simulink model "visual_line_follower_with_debug"  (R2026a)
settings: Solver=FixedStepDiscrete  StopTime=40  FixedStep=MJ_StepTime  EnableMultiTasking=on
InitFcn:
  | run(fullfile(fileparts(get_param(bdroot,"FileName")),"runtime","init","configure_turtlebot3_visual_line_follower_paths.m"));
model workspace (MAT data in the model file):
  BaseLinearSpeed = 5
  BaseSpeedScale = 0.03
  Kd_Line = 0.35
  Ki_Line = 0
  Kp_Line = 5
  LocalPath_CurvatureGain = 0.04
  LocalPath_HeadingGain = 0.35
  LocalPath_LateralGain = 0.6
  LocalPath_LookaheadDistance = 0.2
  LocalPath_NumPoints = 30
  LocalPath_ROIFraction = 0.3
  MJ_StepTime = 0.002
  MJ_TargetLateralPosition = 0
  MaxAngularSpeed = 1.5
  MaxWheelSpeed = 7.9
  N_Line = 20
  OriginBot_ErrorScale = 500
  OriginBot_MaxSaturation = 0.3
  OriginBot_MinBrightness = 70
  OriginBot_MinPixels = 30
  OriginBot_ROIHeight = 45
  OriginBot_ROIStartFraction = 0.72
  SteeringSign = -1
  TB3_WheelRadius = 0.033
  TB3_WheelSeparation = 0.16
  Ts_Control = 0.05
  Ts_Vision = 0.05
  TurtleBot3MuJoCoMap = "complex"
  TurtleBot3MuJoCoScene = ""
values from neighbouring files (symbols this model uses):
  src = get_param(source, "PortHandles")    [add_local_path_to_visual_model.m]
undefined symbols (not defined in the file or in its folder): originbot_line_follower_debug_frame, originbot_sliding_window_path_generator
libraries: mjLib x1, slpidlib x1
settings Model: ExtModeTrigDuration=10000  Creator=HP  LastModifiedBy=kevin
settings SolverCC: PositivePriorityOrder=on
settings ConfigComp: CovMetricSettings=dswe

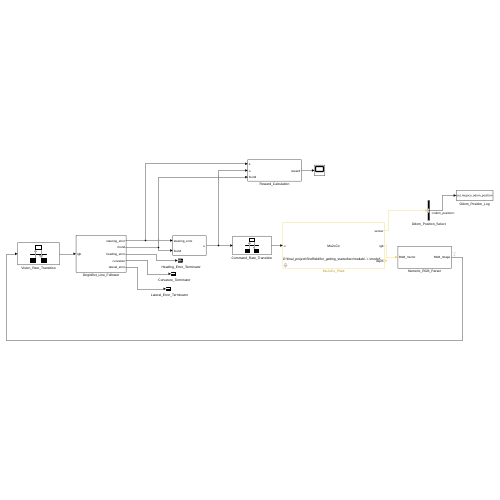
[thumbnail: Simulink's stored preview of the top-level diagram]
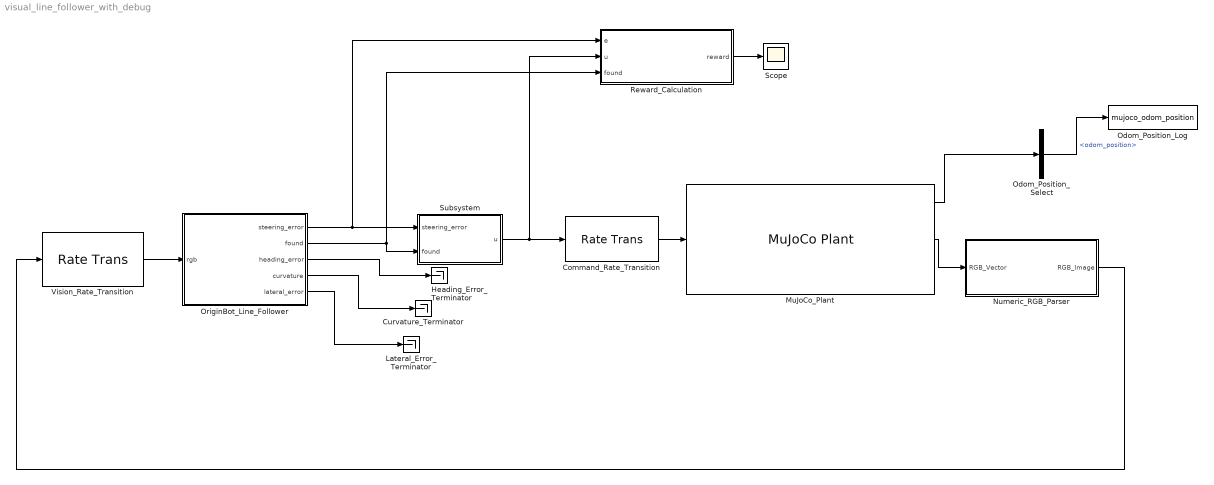
== system visual_line_follower_with_debug ==
  Command_Rate_Transition : RateTransition  OutPortSampleTime=MJ_StepTime
  Curvature_Terminator : Terminator
  Heading_Error_Terminator : Terminator
  Lateral_Error_Terminator : Terminator
  MuJoCo_Plant : mjLib/MuJoCo Plant  controlBus=[]  sensorBus=mj_bus_sensor_7979902499018342666  controlLength=[]  sensorLength=[]  rgbLength=[]  depthLength=[]  sampleTime=0.002  xmlFileRel=D:\final_project\Sheffield\for_getting_started\src\matlab\..\..\model\mujoco\turtlebot3\simple_camera_track_turtlebot3_burger_visual_scene.xml  xmlFile=D:\final_project\Sheffield\for_getting_started\src\matlab\..\..\model\mujoco\turtlebot3\simple_camera_track_turtlebot3_burger_visual_scene.xml  renderingType=Local  vsync=off  visualFPS=60  zoomLevel=1  znear=0.062275  zfar=311.3772  cameraSampleTime=Ts_Vision  rgbOutOption=on  depthOutOption=off  controlInterfaceType=Vector
      settings: SourceProductName=MuJoCo Simulator
  Numeric_RGB_Parser : Subsystem
  Odom_Position_Log : ToWorkspace  VariableName=mujoco_odom_position  SaveFormat=Timeseries  SampleTime=-1
  Odom_Position_Select : BusSelector  OutputSignals=odom_position
  OriginBot_Line_Follower : Subsystem
  Reward_Calculation : Subsystem
  Scope : Scope
      settings: ActiveDisplayYMinimum=-41.521611192700504  ActiveDisplayYMaximum=3.5588120226586528
  Subsystem : Subsystem
  Vision_Rate_Transition : RateTransition  OutPortSampleTime=Ts_Vision
  wires:
  Vision_Rate_Transition/1 -> OriginBot_Line_Follower/1(rgb)
  OriginBot_Line_Follower/1(steering_error) -> Reward_Calculation/1(e), Subsystem/1(steering_error)
  OriginBot_Line_Follower/3(heading_error) -> Heading_Error_Terminator/1
  OriginBot_Line_Follower/2(found) -> Reward_Calculation/3(found), Subsystem/2(found)
  OriginBot_Line_Follower/4(curvature) -> Curvature_Terminator/1
  OriginBot_Line_Follower/5(lateral_error) -> Lateral_Error_Terminator/1
  Subsystem/1(u) -> Reward_Calculation/2(u), Command_Rate_Transition/1
  Reward_Calculation/1(reward) -> Scope/1
  Command_Rate_Transition/1 -> MuJoCo_Plant/1
  MuJoCo_Plant/1 -> Odom_Position_Select/1
  MuJoCo_Plant/2 -> Numeric_RGB_Parser/1(RGB_Vector)
  Odom_Position_Select/1 -> Odom_Position_Log/1  "<odom_position>"
  Numeric_RGB_Parser/1(RGB_Image) -> Vision_Rate_Transition/1

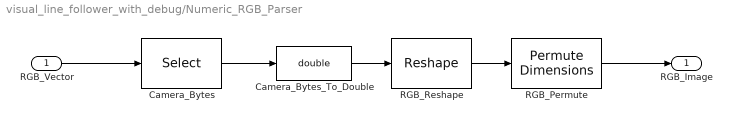
== system visual_line_follower_with_debug/Numeric_RGB_Parser ==
  RGB_Vector : Inport
  Camera_Bytes : Selector  InputPortWidth=921601  IndexOptions=Index vector (dialog)  Indices=1:921600  OutputSizes=1
  Camera_Bytes_To_Double : DataTypeConversion  OutDataTypeStr=double
  RGB_Permute : PermuteDimensions  Order=[3 2 1]
  RGB_Reshape : Reshape  OutputDimensionality=Customize  OutputDimensions=[3,640,480]
  RGB_Image : Outport
  wires:
  Camera_Bytes_To_Double/1 -> RGB_Reshape/1
  RGB_Permute/1 -> RGB_Image/1
  RGB_Reshape/1 -> RGB_Permute/1
  Camera_Bytes/1 -> Camera_Bytes_To_Double/1
  RGB_Vector/1 -> Camera_Bytes/1

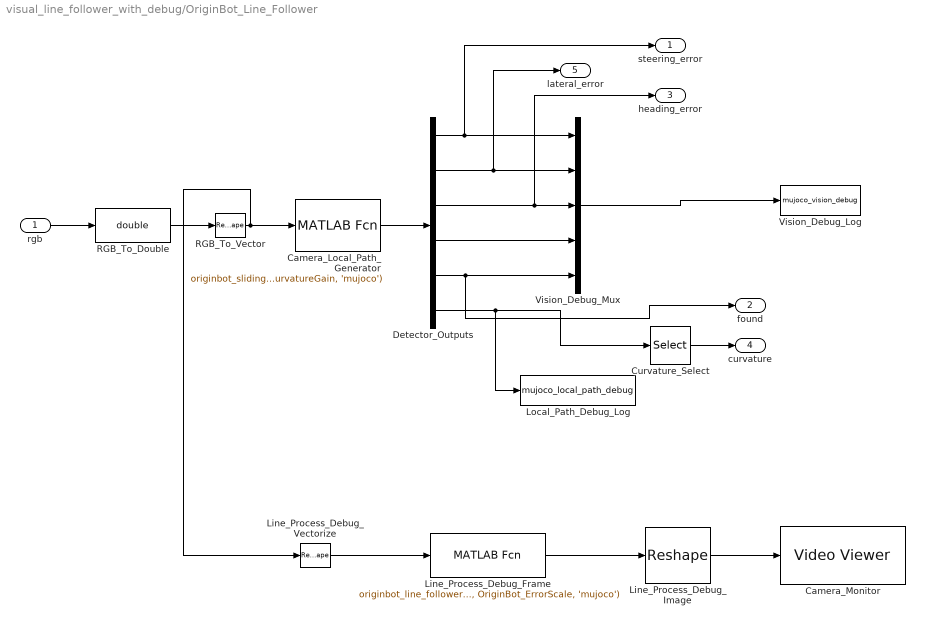
== system visual_line_follower_with_debug/OriginBot_Line_Follower ==
  rgb : Inport
  Camera_Local_Path_Generator : MATLABFcn  MATLABFcn=originbot_sliding_window_path_generator(u, LocalPath_ROIFraction, LocalPath_NumPoints, OriginBot_MinBrightness, OriginBot_MaxSaturation, OriginBot_MinPixels, OriginBot_ErrorScale, LocalPath_LookaheadDistance, LocalPath_LateralGain, LocalPath_HeadingGain, LocalPath_CurvatureGain, 'mujoco')  OutputDimensions=72  OutputSignalType=real  SampleTime=Ts_Vision
  Camera_Monitor : VideoViewer  FigPos=[402 652 810 551]
  Curvature_Select : Selector  InputPortWidth=67  IndexOptions=Index vector (dialog)  Indices=4  OutputSizes=1
  Detector_Outputs : Demux  Outputs=[1 1 1 1 1 67]
  Line_Process_Debug_Frame : MATLABFcn  MATLABFcn=originbot_line_follower_debug_frame(u, LocalPath_ROIFraction, LocalPath_NumPoints, OriginBot_MinBrightness, OriginBot_MaxSaturation, OriginBot_MinPixels, OriginBot_ErrorScale, 'mujoco')
  Line_Process_Debug_Image : Reshape  OutputDimensionality=Customize  OutputDimensions=[480,640,3]
  Line_Process_Debug_Vectorize : Reshape  OutputDimensionality=Column vector (2-D)
  Local_Path_Debug_Log : ToWorkspace  VariableName=mujoco_local_path_debug  SaveFormat=Timeseries  SampleTime=-1
  RGB_To_Double : DataTypeConversion  OutDataTypeStr=double
  RGB_To_Vector : Reshape  OutputDimensionality=Column vector (2-D)
  Vision_Debug_Log : ToWorkspace  VariableName=mujoco_vision_debug  SaveFormat=Timeseries  SampleTime=-1
  Vision_Debug_Mux : Mux  Inputs=5
  steering_error : Outport
  found : Outport  Port=2
  heading_error : Outport  Port=3
  curvature : Outport  Port=4
  lateral_error : Outport  Port=5
  wires:
  Vision_Debug_Mux/1 -> Vision_Debug_Log/1
  Detector_Outputs/1 -> steering_error/1, Vision_Debug_Mux/1
  Detector_Outputs/5 -> Vision_Debug_Mux/5, found/1
  Detector_Outputs/2 -> Vision_Debug_Mux/2, lateral_error/1
  Detector_Outputs/6 -> Curvature_Select/1, Local_Path_Debug_Log/1
  Detector_Outputs/3 -> heading_error/1, Vision_Debug_Mux/3
  Detector_Outputs/4 -> Vision_Debug_Mux/4
  RGB_To_Double/1 -> RGB_To_Vector/1
  RGB_To_Vector/1 -> Camera_Local_Path_Generator/1, Line_Process_Debug_Vectorize/1
  rgb/1 -> RGB_To_Double/1
  Camera_Local_Path_Generator/1 -> Detector_Outputs/1
  Curvature_Select/1 -> curvature/1
  Line_Process_Debug_Frame/1 -> Line_Process_Debug_Image/1
  Line_Process_Debug_Image/1 -> Camera_Monitor/1
  Line_Process_Debug_Vectorize/1 -> Line_Process_Debug_Frame/1

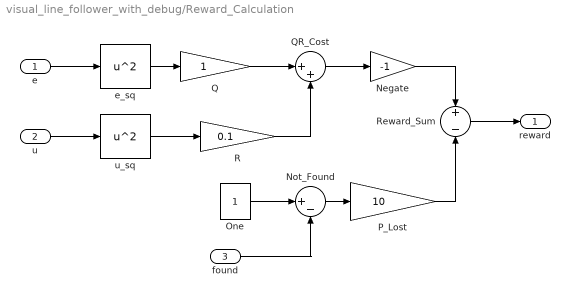
== system visual_line_follower_with_debug/Reward_Calculation ==
  e : Inport
  u : Inport  Port=2
  found : Inport  Port=3
  Negate : Gain  Gain=-1
  Not_Found : Sum  Inputs=|+-
  One : Constant
  P_Lost : Gain  Gain=10
  Q : Gain
  QR_Cost : Sum  Inputs=|++
  R : Gain  Gain=0.1
  Reward_Sum : Sum  Inputs=+-
  e_sq : Math  Operator=square
  u_sq : Math  Operator=square
  reward : Outport
  wires:
  Q/1 -> QR_Cost/1
  e/1 -> e_sq/1
  u/1 -> u_sq/1
  R/1 -> QR_Cost/2
  e_sq/1 -> Q/1
  u_sq/1 -> R/1
  One/1 -> Not_Found/1
  found/1 -> Not_Found/2
  QR_Cost/1 -> Negate/1
  Not_Found/1 -> P_Lost/1
  P_Lost/1 -> Reward_Sum/2
  Negate/1 -> Reward_Sum/1
  Reward_Sum/1 -> reward/1

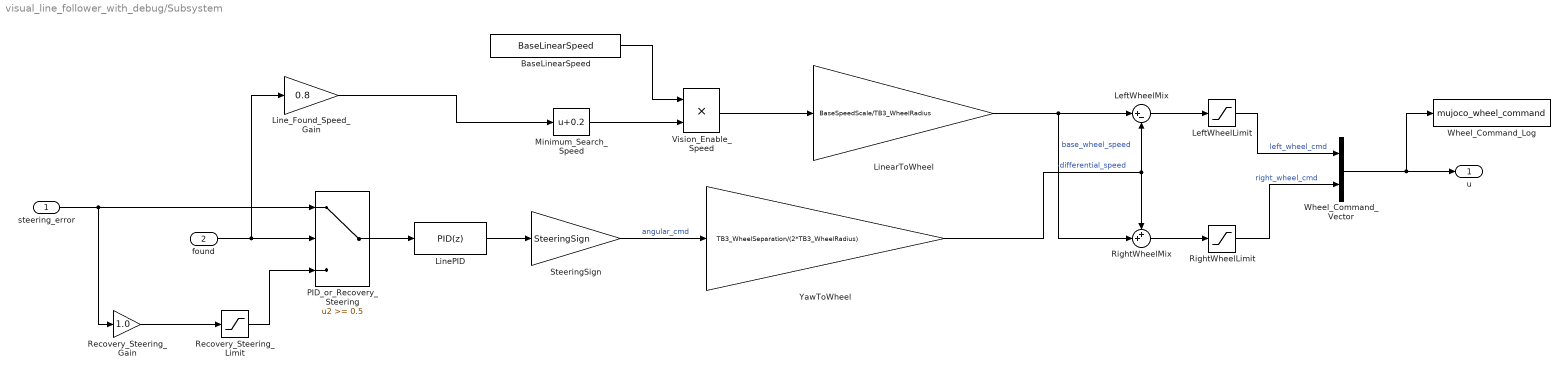
== system visual_line_follower_with_debug/Subsystem ==
  steering_error : Inport
  found : Inport  Port=2
  BaseLinearSpeed : Constant  Value=BaseLinearSpeed
  LeftWheelLimit : Saturate  UpperLimit=MaxWheelSpeed  LowerLimit=-MaxWheelSpeed
  LeftWheelMix : Sum  Inputs=|+-
  LinePID : slpidlib/PID Controller  Controller=PID  Form=Parallel  TimeDomain=Discrete-time  UseExternalTs=off  SampleTime=Ts_Control  IntegratorMethod=Backward Euler  FilterMethod=Trapezoidal  ControllerParametersSource=internal  P=Kp_Line  I=Ki_Line  UseKiTs=off  D=Kd_Line  UseExternalDerivativeSource=off  N=N_Line  UseFilter=on  TunerSelectOption=Transfer Function Based (PID Tuner App)  InitialConditionSource=internal  InitialConditionForIntegrator=0  InitialConditionForFilter=0  DifferentiatorICPrevScaledInput=0  ExternalReset=none  TrackingMode=off  Kt=1  LimitOutput=on  SatLimitsSource=internal  UpperSaturationLimit=MaxAngularSpeed  LowerSaturationLimit=-MaxAngularSpeed  LinearizeAsGain=off  AntiWindupMode=back-calculation  Kb=1  LimitIntegrator=off  UpperIntegratorSaturationLimit=inf  LowerIntegratorSaturationLimit=-inf  POutMin=[]  POutMax=[]  IOutMin=[]  IOutMax=[]  DOutMin=[]  DOutMax=[]  NOutMin=[]  NOutMax=[]  SumOutMin=[]  SumOutMax=[]  SaturationOutMin=[]  SaturationOutMax=[]  PParamMin=[]  PParamMax=[]  IParamMin=[]  IParamMax=[]  DParamMin=[]  DParamMax=[]  NParamMin=[]  NParamMax=[]  KbParamMin=[]  KbParamMax=[]  KtParamMin=[]  KtParamMax=[]  KbOutMin=[]  KbOutMax=[]  KtOutMin=[]  KtOutMax=[]  IntegratorOutMin=[]  IntegratorOutMax=[]  FilterOutMin=[]  FilterOutMax=[]  SumI1OutMin=[]  SumI1OutMax=[]  SumI2OutMin=[]  SumI2OutMax=[]  SumI3OutMin=[]  SumI3OutMax=[]  SumI4OutMin=[]  SumI4OutMax=[]  SumDOutMin=[]  SumDOutMax=[]  DifferentiatorOutMin=[]  DifferentiatorOutMax=[]  FilterDiffOutCoefMin=[]  FilterDiffOutCoefMax=[]  ReciprocalOutMin=[]  ReciprocalOutMax=[]  SumDenOutMin=[]  SumDenOutMax=[]  SumNumOutMin=[]  SumNumOutMax=[]  DivideOutMin=[]  DivideOutMax=[]  UdiffTsProdOutMin=[]  UdiffTsProdOutMax=[]  NTsProdOutMin=[]  NTsProdOutMax=[]  UintegralTsProdOutMin=[]  UintegralTsProdOutMax=[]  UngainTsProdOutMin=[]  UngainTsProdOutMax=[]  ClampingZeroOutDataTypeStr=Inherit: Inherit via back propagation  ClampingZeroOutMin=[]  ClampingZeroOutMax=[]  FilterDenConstantOutDataTypeStr=Inherit: Inherit via back propagation  FilterDenConstantOutMin=[]  FilterDenConstantOutMax=[]  PCopyOutDataTypeStr=Inherit: Inherit via back propagation  PCopyOutMin=[]  PCopyOutMax=[]  NCopyOutDataTypeStr=Inherit: Inherit via back propagation  NCopyOutMin=[]  NCopyOutMax=[]  IntegratorContinuousStateAttributes=''  IntegratorStateMustResolveToSignalObject=off  IntegratorRTWStateStorageClass=Auto  FilterContinuousStateAttributes=''  FilterStateMustResolveToSignalObject=off  FilterRTWStateStorageClass=Auto  ParallelPVariant=InternalParameters  IdealPVariant=Disabled  IVariant=InternalParameters  DVariant=InternalParameters  IntegratorVariant=Discrete  SatVariant=Enabled  AWVariant=BackCalculation  PCopyVariant=Disabled  TRVariant=Disabled  FdbkBlocksVariant=Feedback  IdealPFdbkVariant=Passthrough  SatFdbkVariant=Enabled  DerivativeFilterVariant=TrapezoidalFilter  NVariant=InternalParameters  NCopyVariant=InternalParameters  FilterICVariant=InternalICsFilter  IntegratorICVariant=InternalICs  ExternalResetVariant=Disabled  TRSumVariant=Passthrough  SumFdbkVariant=Enabled  SumVariant=Sum_PID  TsampFilterVariant=InternalTs  TsampNgainVariant=Passthrough  TsampIntegralVariant=Disabled_SignalSpec  ExternalSaturationOutDataTypeStr=Inherit: Same as second input  DerivativeSourceVariant=ErrorSignal  PreIntVariant=InternalPreInt
      settings: LibrarySourceBlock=hdlsllib/Discrete/Discrete PID Controller
  Line_Found_Speed_Gain : Gain  Gain=0.8
  LinearToWheel : Gain  Gain=BaseSpeedScale/TB3_WheelRadius
  Minimum_Search_Speed : Bias  Bias=0.2
  PID_or_Recovery_Steering : Switch  Threshold=0.5
  Recovery_Steering_Gain : Gain  Gain=1.0
  Recovery_Steering_Limit : Saturate  UpperLimit=0.45  LowerLimit=-0.45
  RightWheelLimit : Saturate  UpperLimit=MaxWheelSpeed  LowerLimit=-MaxWheelSpeed
  RightWheelMix : Sum  Inputs=++|
  SteeringSign : Gain  Gain=SteeringSign
  Vision_Enable_Speed : Product  Inputs=**
  Wheel_Command_Log : ToWorkspace  VariableName=mujoco_wheel_command  SaveFormat=Timeseries  SampleTime=-1
  Wheel_Command_Vector : Mux  Inputs=2
  YawToWheel : Gain  Gain=TB3_WheelSeparation/(2*TB3_WheelRadius)
  u : Outport
  wires:
  LeftWheelLimit/1 -> Wheel_Command_Vector/1  "left_wheel_cmd"
  steering_error/1 -> Recovery_Steering_Gain/1, PID_or_Recovery_Steering/1
  Minimum_Search_Speed/1 -> Vision_Enable_Speed/2
  found/1 -> Line_Found_Speed_Gain/1, PID_or_Recovery_Steering/2
  PID_or_Recovery_Steering/1 -> LinePID/1
  Recovery_Steering_Gain/1 -> Recovery_Steering_Limit/1
  Recovery_Steering_Limit/1 -> PID_or_Recovery_Steering/3
  Line_Found_Speed_Gain/1 -> Minimum_Search_Speed/1
  LinePID/1 -> SteeringSign/1
  BaseLinearSpeed/1 -> Vision_Enable_Speed/1
  Vision_Enable_Speed/1 -> LinearToWheel/1
  SteeringSign/1 -> YawToWheel/1  "angular_cmd"
  LinearToWheel/1 -> LeftWheelMix/1, RightWheelMix/2  "base_wheel_speed"
  YawToWheel/1 -> RightWheelMix/1, LeftWheelMix/2  "differential_speed"
  LeftWheelMix/1 -> LeftWheelLimit/1
  RightWheelMix/1 -> RightWheelLimit/1
  RightWheelLimit/1 -> Wheel_Command_Vector/2  "right_wheel_cmd"
  Wheel_Command_Vector/1 -> Wheel_Command_Log/1, u/1
